simulink model "reglersystem"  (R2017a)
settings: Solver=FixedStepAuto  StartTime=0.0  StopTime=inf  RelTol=1e-3
libraries: robotlib x9, simulink x2
settings Model: Creator=simonpersson  LastModifiedBy=simonpersson
settings OptimizationCC: PassReuseOutputArgsAs=Individual arguments  MaxStackSize=64
settings DebuggingCC: ParameterTunabilityLossMsg=error
settings HardwareCC: ProdBitPerPointer=32  ProdBitPerSizeT=32  ProdBitPerPtrDiffT=32  ProdLargestAtomicFloat=None  ProdIntDivRoundTo=Undefined  ProdEndianess=Unspecified  ProdWordSize=32  ProdHWDeviceType=Generic->Unspecified (assume 32-bit Generic)
settings SFSimCC: MATLABDynamicMemAlloc=off
settings RTWCC: SystemTargetFile=ert.tlc  HardwareBoard=Robot Operating System (ROS)  TLCOptions="-aInlineSetEventsForThisBaseRateFcn=TLC_FALSE -aSuppressMultiTaskScheduler=TLC_FALSE  -aRateBasedStepFcn=0"  TemplateMakefile=ert_default_tmf  Description=Embedded Coder  GenerateReport=on  Toolchain=Catkin  IncludeHyperlinkInReport=on  LaunchReport=on  TargetLang=C++  GenerateTraceInfo=on  GenerateTraceReport=on  GenerateTraceReportSl=on  GenerateTraceReportSf=on  GenerateTraceReportEml=on
settings CodeAppCC: ForceParamTrailComments=on  IgnoreCustomStorageClasses=off  OperatorAnnotations=on  SimulinkDataObjDesc=on  SFDataObjDesc=on  MATLABFcnDesc=on  InsertBlockDesc=on  MATLABSourceComments=on
settings ERTTargetCC: SupportContinuousTime=on

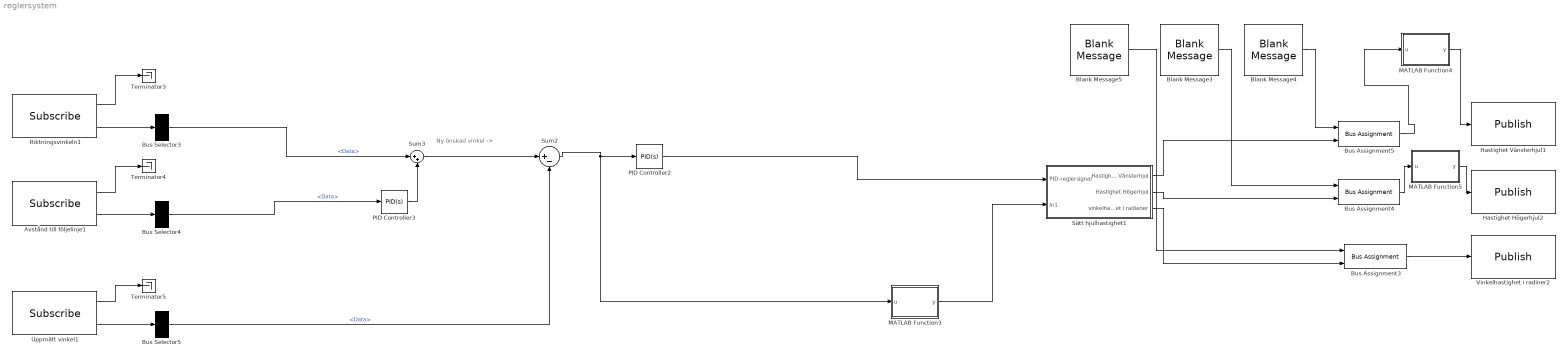
== system reglersystem ==
  note: Ny önskad vinkel ->
  Avstånd till följelinje1 : robotlib/Subscribe  SourceLibraryInfo=This block requires Robotics System Toolbox  topicSource=Specify your own  topic=/distSide_camshifttrack  messageType=std_msgs/Float64  sampleTime=inf  messageQueueLength=1
      settings: SourceProductBaseCode=RO
  Blank Message3 : robotlib/Blank Message  SourceLibraryInfo=This block requires Robotics System Toolbox  messageType=std_msgs/Float64  SampleTime=inf
      settings: SourceProductBaseCode=RO
  Blank Message4 : robotlib/Blank Message  SourceLibraryInfo=This block requires Robotics System Toolbox  messageType=std_msgs/Float64  SampleTime=inf
      settings: SourceProductBaseCode=RO
  Blank Message5 : robotlib/Blank Message  SourceLibraryInfo=This block requires Robotics System Toolbox  messageType=std_msgs/Float64  SampleTime=inf
      settings: SourceProductBaseCode=RO
  Bus Assignment3 : BusAssignment  AssignedSignals=Data
  Bus Assignment4 : BusAssignment  AssignedSignals=Data
  Bus Assignment5 : BusAssignment  AssignedSignals=Data
  Bus Selector3 : BusSelector  OutputSignals=Data
  Bus Selector4 : BusSelector  OutputSignals=Data
  Bus Selector5 : BusSelector  OutputSignals=Data
  Hastighet Högerhjul2 : robotlib/Publish  SourceLibraryInfo=This block requires Robotics System Toolbox  topicSource=Specify your own  topic=/motor_H  messageType=std_msgs/Float64  messageQueueLength=1
      settings: SourceProductBaseCode=RO
  Hastighet Vänsterhjul1 : robotlib/Publish  SourceLibraryInfo=This block requires Robotics System Toolbox  topicSource=Specify your own  topic=/motor_V  messageType=std_msgs/Float64  messageQueueLength=1
      settings: SourceProductBaseCode=RO
  MATLAB Function3 : MATLAB Function  TreatAsAtomicUnit=on
  MATLAB Function4 : MATLAB Function  TreatAsAtomicUnit=on
  MATLAB Function5 : MATLAB Function  TreatAsAtomicUnit=on
  PID Controller2 : simulink/Continuous/PID Controller  Controller=PID  TimeDomain=Continuous-time  SampleTime=-1  IntegratorMethod=Forward Euler  FilterMethod=Forward Euler  Form=Parallel  UseFilter=on  ControllerParametersSource=internal  P=0.367924650540206  I=0.00322808256007609  D=0.282931123087523  N=10.589930050352  InitialConditionSource=internal  InitialConditionForIntegrator=0  InitialConditionForFilter=0  ExternalReset=none  LimitOutput=off  UpperSaturationLimit=inf  LowerSaturationLimit=-inf  LinearizeAsGain=on  AntiWindupMode=none  Kb=1  TrackingMode=off  Kt=1  PParamMin=[]  PParamMax=[]  IParamMin=[]  IParamMax=[]  DParamMin=[]  DParamMax=[]  NParamMin=[]  NParamMax=[]  KbParamMin=[]  KbParamMax=[]  KtParamMin=[]  KtParamMax=[]  POutMin=[]  POutMax=[]  IOutMin=[]  IOutMax=[]  DOutMin=[]  DOutMax=[]  NOutMin=[]  NOutMax=[]  KbOutMin=[]  KbOutMax=[]  KtOutMin=[]  KtOutMax=[]  IntegratorOutMin=[]  IntegratorOutMax=[]  FilterOutMin=[]  FilterOutMax=[]  SumOutMin=[]  SumOutMax=[]  SumI1OutMin=[]  SumI1OutMax=[]  SumI2OutMin=[]  SumI2OutMax=[]  SumI3OutMin=[]  SumI3OutMax=[]  SumDOutMin=[]  SumDOutMax=[]  SaturationOutMin=[]  SaturationOutMax=[]  IntegratorContinuousStateAttributes=''  IntegratorStateMustResolveToSignalObject=off  IntegratorRTWStateStorageClass=Auto  FilterContinuousStateAttributes=''  FilterStateMustResolveToSignalObject=off  FilterRTWStateStorageClass=Auto  DifferentiatorICPrevScaledInput=0  DifferentiatorOutMin=[]  DifferentiatorOutMax=[]  InitialConditionSetting=State (most efficient)
  PID Controller3 : simulink/Continuous/PID Controller  Controller=PID  TimeDomain=Continuous-time  SampleTime=-1  IntegratorMethod=Forward Euler  FilterMethod=Forward Euler  Form=Parallel  UseFilter=on  ControllerParametersSource=internal  P=-0.83587508070568  I=-0.105426269945514  D=-0.832310320830903  N=2.97524164324084  InitialConditionSource=internal  InitialConditionForIntegrator=0  InitialConditionForFilter=0  ExternalReset=none  LimitOutput=off  UpperSaturationLimit=inf  LowerSaturationLimit=-inf  LinearizeAsGain=on  AntiWindupMode=none  Kb=1  TrackingMode=off  Kt=1  PParamMin=[]  PParamMax=[]  IParamMin=[]  IParamMax=[]  DParamMin=[]  DParamMax=[]  NParamMin=[]  NParamMax=[]  KbParamMin=[]  KbParamMax=[]  KtParamMin=[]  KtParamMax=[]  POutMin=[]  POutMax=[]  IOutMin=[]  IOutMax=[]  DOutMin=[]  DOutMax=[]  NOutMin=[]  NOutMax=[]  KbOutMin=[]  KbOutMax=[]  KtOutMin=[]  KtOutMax=[]  IntegratorOutMin=[]  IntegratorOutMax=[]  FilterOutMin=[]  FilterOutMax=[]  SumOutMin=[]  SumOutMax=[]  SumI1OutMin=[]  SumI1OutMax=[]  SumI2OutMin=[]  SumI2OutMax=[]  SumI3OutMin=[]  SumI3OutMax=[]  SumDOutMin=[]  SumDOutMax=[]  SaturationOutMin=[]  SaturationOutMax=[]  IntegratorContinuousStateAttributes=''  IntegratorStateMustResolveToSignalObject=off  IntegratorRTWStateStorageClass=Auto  FilterContinuousStateAttributes=''  FilterStateMustResolveToSignalObject=off  FilterRTWStateStorageClass=Auto  DifferentiatorICPrevScaledInput=0  DifferentiatorOutMin=[]  DifferentiatorOutMax=[]  InitialConditionSetting=State (most efficient)
  Riktningsvinkeln1 : robotlib/Subscribe  SourceLibraryInfo=This block requires Robotics System Toolbox  topicSource=Specify your own  topic=/ang__camshifttrack  messageType=std_msgs/Float64  sampleTime=inf  messageQueueLength=1
      settings: SourceProductBaseCode=RO
  Sum2 : Sum  Inputs=|+-
  Sum3 : Sum  Inputs=|++
  Sätt hjulhastighet1 : Subsystem
  Terminator3 : Terminator
  Terminator4 : Terminator
  Terminator5 : Terminator
  Uppmätt vinkel1 : robotlib/Subscribe  SourceLibraryInfo=This block requires Robotics System Toolbox  topicSource=Specify your own  topic=/heading  messageType=std_msgs/Float64  sampleTime=inf  messageQueueLength=1
      settings: SourceProductBaseCode=RO
  Vinkelhastighet i radiner2 : robotlib/Publish  SourceLibraryInfo=This block requires Robotics System Toolbox  topicSource=Specify your own  topic=/vinkelHastighet  messageType=std_msgs/Float64  messageQueueLength=1
      settings: SourceProductBaseCode=RO
  wires:
  MATLAB Function3/1(y) -> Sätt hjulhastighet1/2(In1)
  PID Controller3/1 -> Sum3/2
  Sum3/1 -> Sum2/1
  PID Controller2/1 -> Sätt hjulhastighet1/1("PID-reglersignal ")
  Sum2/1 -> PID Controller2/1, MATLAB Function3/1(u)
  Riktningsvinkeln1/2 -> Bus Selector3/1
  Bus Selector3/1 -> Sum3/1  "<Data>"
  Riktningsvinkeln1/1 -> Terminator3/1
  Avstånd till följelinje1/1 -> Terminator4/1
  Bus Selector4/1 -> PID Controller3/1  "<Data>"
  Avstånd till följelinje1/2 -> Bus Selector4/1
  Bus Selector5/1 -> Sum2/2  "<Data>"
  Uppmätt vinkel1/2 -> Bus Selector5/1
  Uppmätt vinkel1/1 -> Terminator5/1
  Bus Assignment5/1 -> MATLAB Function4/1(u)
  MATLAB Function5/1(y) -> Hastighet Högerhjul2/1
  Bus Assignment3/1 -> Vinkelhastighet i radiner2/1
  Sätt hjulhastighet1/2(Hastighet Högerhjul) -> Bus Assignment4/2
  Bus Assignment4/1 -> MATLAB Function5/1(u)
  Blank Message3/1 -> Bus Assignment4/1
  Blank Message4/1 -> Bus Assignment5/1
  Blank Message5/1 -> Bus Assignment3/1
  Sätt hjulhastighet1/3(vinkelhastighet i radianer) -> Bus Assignment3/2
  Sätt hjulhastighet1/1(Hastighet Vänsterhjul) -> Bus Assignment5/2
  MATLAB Function4/1(y) -> Hastighet Vänsterhjul1/1

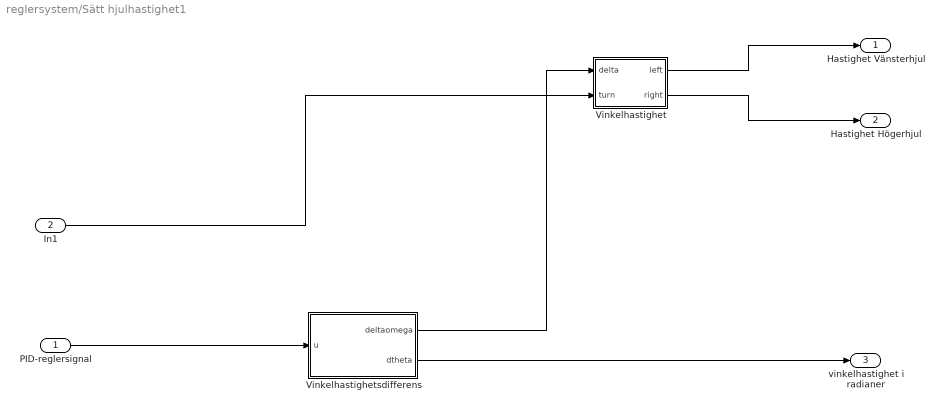
== system reglersystem/Sätt hjulhastighet1 ==
  "PID-reglersignal " : Inport
  In1 : Inport  Port=2
  Vinkelhastighet : MATLAB Function  TreatAsAtomicUnit=on
  Vinkelhastighetsdifferens : MATLAB Function  TreatAsAtomicUnit=on
  Hastighet Vänsterhjul : Outport
  Hastighet Högerhjul : Outport  Port=2
  vinkelhastighet i radianer : Outport  Port=3
  wires:
  "PID-reglersignal "/1 -> Vinkelhastighetsdifferens/1(u)
  Vinkelhastighetsdifferens/1(deltaomega) -> Vinkelhastighet/1(delta)
  Vinkelhastighetsdifferens/2(dtheta) -> vinkelhastighet i radianer/1
  Vinkelhastighet/1(left) -> Hastighet Vänsterhjul/1
  Vinkelhastighet/2(right) -> Hastighet Högerhjul/1
  In1/1 -> Vinkelhastighet/2(turn)

== matlab function reglersystem/MATLAB Function3 ==
  data: u input; y output
function y = fcn(u)
%#codegen
vinkelgrans=0.7;
if(u>vinkelgrans)
    u=1;
else if(u<-vinkelgrans)
        u=-1;
else
    u=0;
    end
end

y = u;

== matlab function reglersystem/Sätt hjulhastighet1/Vinkelhastighet ==
  data: delta input; left output; right output; turn input
function [left,right] = fcn(delta,turn)
r=0.075;
if(turn==0)
if(delta<0)%sväng höger
    left=(1/(2*r*pi))*2*pi;
    right=((1/(2*r*pi))*2*pi)-abs(delta);
  if(right<0)
      right=0;
    end
else if(delta>0)%sväng vänster
    right=(1/(2*r*pi))*2*pi;
    left=((1/(2*r*pi))*2*pi)-abs(delta); 
    if(left<0)
        left=0;
    end
else % kör rakt
    right =(1/(2*r*pi))*2*pi;
    left=(1/(2*r*pi))*2*pi;
    end
end
else if(turn<0)  
    right =(1/(6*r*pi))*2*pi;
    left=-(1/(6*r*pi))*2*pi;
    
    else
        right =-(1/(6*r*pi))*2*pi;
        left=(1/(6*r*pi))*2*pi;
    end
end
end

== matlab function reglersystem/Sätt hjulhastighet1/Vinkelhastighetsdifferens ==
  data: u input; deltaomega output; dtheta output
function [deltaomega,dtheta] = fcn(u)
b=0.55; %avstånd mellan hjul
r=0.075; %hjulradie
u=u*360/(2*pi);
z=u;

dtheta=z*2*pi/360;           %robotens vinkelhastighet
deltaomega=((dtheta.*b)./r);         %differensen i vinkelhastighet mellan hjulen
end

== matlab function reglersystem/MATLAB Function4 ==
  data: u input; y output
function y = fcn(u)
y = 11.4474+5.96269 * u;

== matlab function reglersystem/MATLAB Function5 ==
  data: u input; y output
function y = fcn(u)
y = 10.2732+5.41462 * u;
